simulink model "sim81"  (R2017a)
settings: Solver=ode5  StartTime=0.0  StopTime=20  FixedStep=0.001  MaxStep=0.05  RelTol=1e-3
libraries: simulink x1
settings Model: Creator=asus  LastModifiedBy=Lenovo

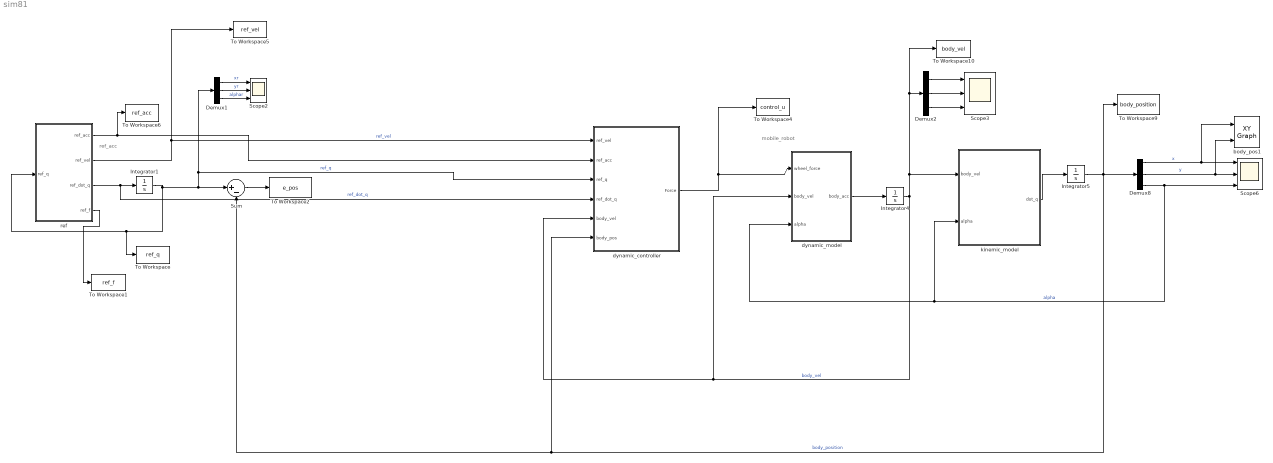
== system sim81 ==
  note: ref_acc
  note: mobile_robot
  Demux1 : Demux  Outputs=3
  Demux2 : Demux  Outputs=3
  Demux8 : Demux  Outputs=3
  Integrator1 : Integrator  InitialCondition=[0;0;pi/4]
  Integrator4 : Integrator  InitialCondition=[0.1 0.1 0.1]  IgnoreLimit=on
  Integrator5 : Integrator  InitialCondition=[2 -2 pi/2]  IgnoreLimit=on
  Scope2 : Scope  NumInputPorts=3
  Scope3 : Scope  NumInputPorts=3
  Scope6 : Scope  NumInputPorts=3
  Sum : Sum  Inputs=|+-
  To Workspace : ToWorkspace  VariableName=ref_q  SampleTime=-1
  To Workspace1 : ToWorkspace  VariableName=ref_f  SampleTime=-1
  To Workspace10 : ToWorkspace  VariableName=body_vel  SampleTime=-1
  To Workspace2 : ToWorkspace  VariableName=e_pos  SampleTime=-1
  To Workspace4 : ToWorkspace  VariableName=control_u  SampleTime=-1
  To Workspace5 : ToWorkspace  VariableName=ref_vel  SampleTime=-1
  To Workspace6 : ToWorkspace  VariableName=ref_acc  SampleTime=-1
  To Workspace9 : ToWorkspace  VariableName=body_position  SampleTime=-1
  body_pos1 : simulink/Sinks/XY Graph  xmin=-10  xmax=10  ymin=-10  ymax=10  st=-1
  dynamic_controller : MATLAB Function  TreatAsAtomicUnit=on
  dynamic_model : MATLAB Function  TreatAsAtomicUnit=on
  kinemic_model : MATLAB Function  TreatAsAtomicUnit=on
  ref : MATLAB Function  TreatAsAtomicUnit=on
  wires:
  Demux1/3 -> Scope2/3  "alphar"
  Demux1/1 -> Scope2/1  "xr"
  Demux1/2 -> Scope2/2  "yr"
  Integrator1/1 -> ref/1(ref_q), To Workspace/1, dynamic_controller/3(ref_q), Demux1/1, Sum/1  "ref_q"
  ref/2(ref_vel) -> dynamic_controller/1(ref_vel), To Workspace5/1  "ref_vel"
  ref/3(ref_dot_q) -> dynamic_controller/4(ref_dot_q), Integrator1/1  "ref_dot_q"
  Demux2/1 -> Scope3/1
  Demux2/2 -> Scope3/2
  Demux2/3 -> Scope3/3
  Demux8/1 -> body_pos1/1, Scope6/1  "x"
  Demux8/2 -> body_pos1/2, Scope6/2  "y"
  Demux8/3 -> dynamic_model/3(alpha), kinemic_model/2(alpha), Scope6/3  "alpha"
  Integrator4/1 -> dynamic_model/2(body_vel), dynamic_controller/5(body_vel), kinemic_model/1(body_vel), To Workspace10/1, Demux2/1  "body_vel"
  dynamic_model/1(body_acc) -> Integrator4/1
  kinemic_model/1(dot_q) -> Integrator5/1
  Integrator5/1 -> dynamic_controller/6(body_pos), Sum/2, To Workspace9/1, Demux8/1  "body_position"
  ref/1(ref_acc) -> To Workspace6/1, dynamic_controller/2(ref_acc)
  Sum/1 -> To Workspace2/1
  dynamic_controller/1(Force) -> dynamic_model/1(wheel_force), To Workspace4/1
  ref/4(ref_f) -> To Workspace1/1

== matlab function sim81/ref ==
  data: ref_q input; ref_acc output; ref_vel output; ref_dot_q output; ref_f output
function [ref_acc,ref_vel, ref_dot_q,ref_f]  = fcn(ref_q)
xr=ref_q(1);
yr=ref_q(2);
alphar=ref_q(3);

axro=0;
ayro=0;
aomegaro=0;

dot_vxr=axro;
dot_vyr=ayro;
dot_omegar=aomegaro;
ref_acc=[dot_vxr;dot_vyr;dot_omegar]; %车体坐标系下 车的参考加速度

vxr=1;
vyr=0;
omegar=0.5;
ref_vel=[vxr;vyr;omegar]; %车体坐标系下的车的参考速度

dotx = vxr*cos(alphar) - vyr*sin(alphar);
doty = vxr*sin(alphar) + vyr*sin(alphar);
dotalpha = omegar;
ref_dot_q=[dotx;doty;dotalpha]; % 世界坐标系下的各轴的速度

ref_f=[0 ; 0];

end

== matlab function sim81/dynamic_model ==
  data: wheel_force input; body_acc output; body_vel input; alpha input
function body_acc = fcn(wheel_force,body_vel,alpha)
%车辆参数
d = 0.18;
l = 0.16;

m = 24;
Iz = 11.89;

c_wheel = 513.6 ; %侧偏刚度
gravity=[0 0 9.81];



FX1 = wheel_force(1);    % 将得到的车轮挂钩牵引力分配
FX2 = wheel_force(2);

vx=body_vel(1);
vy=body_vel(2);
omega=body_vel(3);

beta1=atan( ( vy+l*omega )/( vx+0.000000000000001 ));
beta2=atan( ( vy+l*omega )/( vx+0.000000000000001 ));

FY1=-c_wheel*beta1;
FY2=-c_wheel*beta2;

dot_vx = ( FX1+FX2 )/m + vy*omega;
dot_vy = ( FY1+FY2 )/m - vx*omega;
dot_omega = ( d*(FX2-FX1)- l*(FY1+FY2) )/Iz;

body_acc=[dot_vx ; dot_vy ; dot_omega]; %得到车辆的加速度

% B1=(1/2)*[1 0 -1/d; 
%           1 0 1/d]
% M=[m 0 0
%    0 m 0
%    0 0 I_z]
% 
% V=[0 -m*d_alpha 0;
%    m*d_alpha 0 0;
%     0 0 0]
% G=[m*gravity(3)*sin(gamma)*sin(alpha)
%    m*gravity(3)*sin(gamma)*cos(alpha)
%    0]
% B=(1/wheel_radius)*[1 1;0 0 ;-d d]
% A=[0 1 0]'
% 
% 
% Lambda=Fy1+Fy2+Fy3+Fy4
% 
% kesi=0;
end

== matlab function sim81/dynamic_controller ==
  data: ref_vel input; ref_acc input; ref_q input; ref_dot_q input; Force output; body_vel input; body_pos input
function Force = SMC_controller(ref_vel,ref_acc,ref_q, ref_dot_q,body_vel,body_pos)
%% 参数测试
% ref_vel=[1; 0; 0.5];
% ref_acc=[0 ;0;0];
% ref_q=[0 ;0;pi/4];
% ref_dot_q=[0.5;0.5;0.5];
% body_vel=[0.01 ; 0 ;0];
% body_pos=[2; 2; pi/2];

%%
m = 24;
Iz = 11.89;     l = 0.16;   d = 0.18;
c=[1 0 0; 0 1 0; 0 0 10];    c_wheel = 513.6 ; %侧偏刚度

vx = body_vel(1);
vy = body_vel(2);
omega = body_vel(3);

alpha = body_pos(3);

alphar = ref_q(3);

M=[m 0 0;
   0 m 0;
   0 0 Iz];

R=[cos(alpha) -sin(alpha) 0;
   sin(alpha) cos(alpha) 0;
   0 0 1];

Rr=[cos(alphar) -sin(alphar) 0;
   sin(alphar) cos(alphar) 0;
   0 0 1];
V=[-m*omega*vy;
   m*omega*vx;
   0 ];
A=[0 1 0];

% B=[1 1;0 0; -d d]

B_=1/2*[1 0 -1/d;1 0 1/d];

e_q = body_pos-ref_q;
e_vel = body_vel-ref_vel;

S=c*e_q+e_vel;


beta1=atan( ( vy+l*omega )/( vx ));
beta2=atan( ( vy+l*omega )/( vx ));
% beta1=atan( ( vy+l*omega )/( vx+0.000000000000001 ));
% beta2=atan( ( vy+l*omega )/( vx+0.000000000000001 ));

FY1=-c_wheel*beta1;
FY2=-c_wheel*beta2;

lambda=FY1+FY2;

kesi = 0.25; K=0.165;

% slaw = -kesi*sign(S);     %等速趋近律 kesi>0
slaw = -kesi*sign(S)-K*S;   %指数趋近律 kesi>0   k>0
% slaw = -K*abs(S)^a*sign(S); %幂次趋近律 K>0  1>a>0
u=B_*M*slaw - B_*M*c*R*body_vel + B_*M*Rr*ref_vel-B_*A'*lambda+B_*V+B_*M*ref_acc;

Force=u;



% vxr=ref_vel(1);
% vyr=ref_vel(2);
% omegar=ref_vel(3);
% 
% dot_vxr=ref_acc(1);
% dot_vyr=ref_acc(2);
% dot_omegar=ref_acc(3);
% 
% e_x=e(1);
% e_y=e(2);
% e_alpha=e(3);
% 
% vxa=vel_a(1);
% vya=vel_a(2);
% omegaa=vel_a(3);
% 
% % vx=vxr*cos(e_alpha)+k1*e_x;
% % vy=0;
% % omega=omegar+k2*vxr*e_y+k3*vxr*sin(e_alpha);
% % omega=omegar+k2*vxr*sin(e_alpha)/e_alpha*e_y+k3*e_alpha;
% s1=e_x;
% s2=e_alpha+atan(vxr*e_y);
% 
% 
% ddvr=e_y*dot_vxr/(1+(vxr*e_y)^2);
% % ddey=vxr*dot_e_y/(1+(vxr*e_y)^2);
% fenmu=1/(1+(vxr*e_y)^2);
% 
% 
% kesi1=0.55;
% kesi2=0.55;
% 
% 
% vx=e_y*omegaa+vxr*cos(e_alpha)+kesi1*sign(s1);
% 
% vy=0;
% 
% omega=( omegar + ddvr + fenmu*(vxr*vxr*sin(e_alpha))+kesi2*sign(s2) )/( 1+(vxr*e_x)/(1+(vxr*e_y)^2) )
% 
% 
% 
% 
% v=[vx;vy;omega]
end

== matlab function sim81/kinemic_model ==
  data: body_vel input; dot_q output; alpha input
% body_vel传进来的是【v w】

function dot_q   = fcn(body_vel,alpha)

wheel_radius = 0.330/2;
d = 0.18;
l = 0.16;

R = [cos(alpha) -sin(alpha) 0;
     sin(alpha) cos(alpha) 0;
     0 0 1];
% R_w2v =(wheel_radius).*[1/2     1/2;
%                             0           0;
%                         -1/(2*d)  1/(2*d)];
%                     
% max=1/wheel_radius;
% for i=1:size(wheel_omega,2)
%     if wheel_omega(i)>max
%         wheel_omega(i) = max;
%     else
%         if wheel_omega(i)<-max
%             wheel_omega(i) = -max;
%         else
%             wheel_omega(i) = wheel_omega(i);
%         end
%     end
% end
%  wheel_omega;
                    
                    
                    
% body_vel=R_w2v*wheel_omega; % 本体坐标系下的速度

dot_q = R *body_vel; % 世界坐标系下的速度



end
